simulink model "P1_Sim_2_1"  (R2021a)
settings: Solver=ode5  StartTime=0  StopTime=t  FixedStep=0.01  RelTol=1e-3  AbsTol=1e-6
model workspace (MAT data in the model file):
  socvcb = containers.Map
  socvcb.serialization.keys = {}
  socvcb.serialization.values = {}
  socvcb.serialization.uniformity = 0
  socvcb.serialization.keyType = 'double'
  socvcb.serialization.valueType = 'any'
values from neighbouring files (symbols this model uses):
  amplitude = 0.7    [control.m]
  g = 9.81    [control.m]
  gamma2 = 0.267534    [control.m]
  init_cond = [0 pi/30 0 0]    [control.m]
  K = lqr(A,B,Q,R)    [control.m]
  l = 0.512166    [control.m]
  M = 0.5723    [control.m]
  m = 0.12    [control.m]
  stab_point = [0 0 0 0]    [control.m]
libraries: simulink x12, pid_lib x3, simulink_extras x1
settings Model: ExtModeTrigDuration=18000  ExtModeTrigLevel=0.400000  Creator=jims  LastModifiedBy=Piotr
settings SolverCC: AutoScaleAbsTol=off  AlgebraicLoopSolver=TrustRegion
settings DataIOCC: ExternalInput=[]  InitialState=[]  MaxDataPoints=5000  SaveFormat=StructureWithTime  SignalLoggingSaveFormat=ModelDataLogs  SaveOutput=off  SaveTime=off  ReturnWorkspaceOutputs=off
settings OptimizationCC: BlockReduction=off  BooleanDataType=off  BufferReuse=off  ExpressionDepthLimit=2147483647
settings DebuggingCC: AlgebraicLoopMsg=none  SaveWithParameterizedLinksMsg=none  UnderspecifiedInitializationDetection=Classic  MergeDetectMultiDrivingBlocksExec=none  SignalResolutionControl=TryResolveAllWithWarning  MultiTaskDSMMsg=warning  MultiTaskCondExecSysMsg=none  IntegerOverflowMsg=none  FcnCallInpInsideContextMsg=warning  UnconnectedInputMsg=none  UnconnectedOutputMsg=none  UnconnectedLineMsg=none  StateNameClashWarn=warning  SFUnexpectedBacktrackingDiag=warning  SFNoUnconditionalDefaultTransitionDiag=warning  SFExecutionAtInitializationDiag=none  SFMachineParentedDataDiag=warning  IntegerSaturationMsg=none  ArithmeticOperatorsInVariantConditions=warning
settings HardwareCC: TargetBitPerLong=64  TargetBitPerPointer=64  TargetIntDivRoundTo=Zero  TargetEndianess=LittleEndian  TargetWordSize=64  TargetHWDeviceType=Intel->x86-64
settings ModelReferenceCC: PropagateSignalLabelsOutOfModel=off
settings SFSimCC: SimUseLocalCustomCode=off  CustomCodeUndefinedFunction=UseInterfaceOnly
settings RTWCC: Description=Generic Real-Time Target  RTWUseLocalCustomCode=off  RTWCompilerOptimization=on
settings CodeAppCC: MaxIdLength=95  StateflowObjectComments=on
settings GRTTargetCC: TargetLangStandard=C89/C90 (ANSI)
settings ConfigComp: CovMetricSettings=dw  CovSaveCumulativeToWorkspaceVar=on  CovSaveSingleToWorkspaceVar=on  CovExternalEMLEnable=off  CovSFcnEnable=off

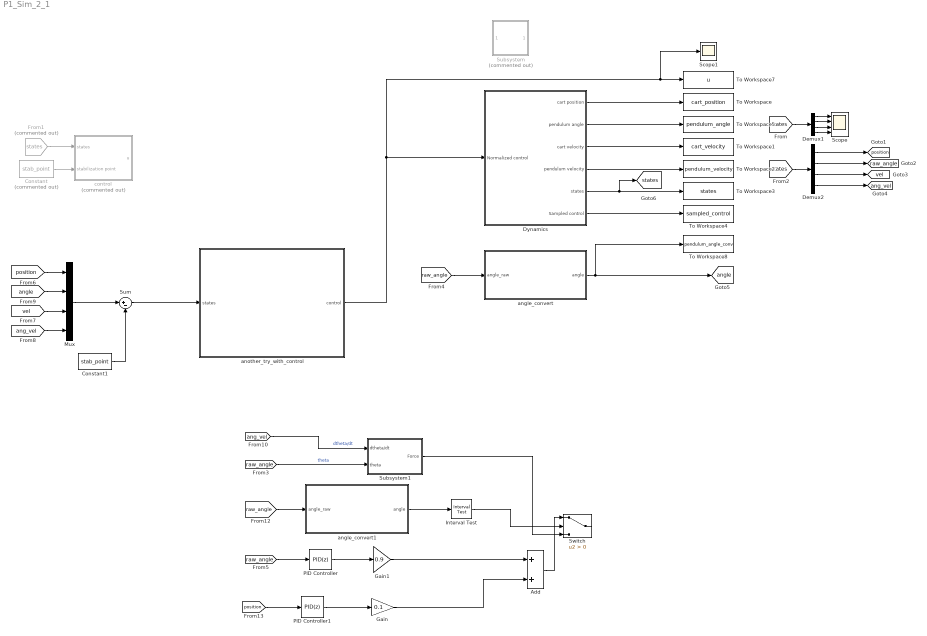
== system P1_Sim_2_1 ==
  Add : Sum
  Constant : Constant  Commented=on  Value=stab_point  OutDataTypeStr=Inherit: Inherit via back propagation
  Constant1 : Constant  Value=stab_point  OutDataTypeStr=Inherit: Inherit via back propagation
  Demux1 : Demux
  Demux2 : Demux
  Dynamics : Subsystem  mask(Dynamics){x_ini=init_cond, m=[0.5723, 0.12], fr=[0.00027344,  1.1975875,  0.5], P4=[0.01955717, 0.0038583, 9.81], Up=[ 12.86, 0.093125], DZ=[0.1, 1.5]}
      mask prompts: x_ini "Initial state vector [x1(0)  x2(0)  x3(0)  x4(0)]"; m "mass of cart (mc)  mass of pendulum (mp)"; fr "friction :  fp  FS  FC"; P4 "Distance (l), Total Inertia moment (J), gravity (g)"; Up "control : magnitude (M)    DZu"; DZ "minimal velocities : cart (DZcv)  pendulum (DZcp)"
      mask help:
      | Pendulum-Cart Dynamics
      |
      | Copyright INTECO 1997
      mask init:
      | DZcv=DZ(1);DZcp=DZ(2);DZu=Up(2);l=P4(1);J=P4(2);g=P4(3);M=Up(1);mc=m(1);mp=m(2);fp=fr(1);FS=fr(2);FC=fr(3);mi=l*(mc+mp);a=l*l+J/(mc+mp);
      mask Display: plot(0,0,100,100,[40,48,48,40,40],[60,60,49,49,60],[37,44],[9,54],[100,8,4,1,0,100,100,0,40,100,100,0,0,40],[44,44,44,44,45,46,45,44,45,45,43,43,46,46],[100,48],[55,55],[0,40],[55,55])
  From1 : From  Commented=on  GotoTag=states  TagVisibility=global
  Gain : Gain  Gain=0.1
  Gain1 : Gain  Gain=0.9
  Interval Test : simulink/Logic and Bit Operations/Interval Test  IntervalClosedRight=on  uplimit=0.5  IntervalClosedLeft=on  lowlimit=-0.5  OutDataTypeStr=boolean
  Mux : Mux
  PID Controller : pid_lib/PID Controller  Controller=PID  Form=Parallel  TimeDomain=Discrete-time  UseExternalTs=off  SampleTime=-1  IntegratorMethod=Forward Euler  FilterMethod=Forward Euler  ControllerParametersSource=internal  P=100  I=1  D=20  UseFilter=on  N=100  TunerSelectOption=Transfer Function Based (PID Tuner App)  InitialConditionSource=internal  InitialConditionForIntegrator=0  InitialConditionForFilter=0  DifferentiatorICPrevScaledInput=0  ExternalReset=none  TrackingMode=off  Kt=1  LimitOutput=off  SatLimitsSource=internal  UpperSaturationLimit=inf  LowerSaturationLimit=-inf  LinearizeAsGain=on  AntiWindupMode=none  Kb=1  POutMin=[]  POutMax=[]  IOutMin=[]  IOutMax=[]  DOutMin=[]  DOutMax=[]  NOutMin=[]  NOutMax=[]  SumOutMin=[]  SumOutMax=[]  SaturationOutMin=[]  SaturationOutMax=[]  PParamMin=[]  PParamMax=[]  IParamMin=[]  IParamMax=[]  DParamMin=[]  DParamMax=[]  NParamMin=[]  NParamMax=[]  KbParamMin=[]  KbParamMax=[]  KtParamMin=[]  KtParamMax=[]  KbOutMin=[]  KbOutMax=[]  KtOutMin=[]  KtOutMax=[]  IntegratorOutMin=[]  IntegratorOutMax=[]  FilterOutMin=[]  FilterOutMax=[]  SumI1OutMin=[]  SumI1OutMax=[]  SumI2OutMin=[]  SumI2OutMax=[]  SumI3OutMin=[]  SumI3OutMax=[]  SumI4OutMin=[]  SumI4OutMax=[]  SumDOutMin=[]  SumDOutMax=[]  DifferentiatorOutMin=[]  DifferentiatorOutMax=[]  FilterDiffOutCoefMin=[]  FilterDiffOutCoefMax=[]  ReciprocalOutMin=[]  ReciprocalOutMax=[]  SumDenOutMin=[]  SumDenOutMax=[]  SumNumOutMin=[]  SumNumOutMax=[]  DivideOutMin=[]  DivideOutMax=[]  UdiffTsProdOutMin=[]  UdiffTsProdOutMax=[]  NTsProdOutMin=[]  NTsProdOutMax=[]  UintegralTsProdOutMin=[]  UintegralTsProdOutMax=[]  UngainTsProdOutMin=[]  UngainTsProdOutMax=[]  IntegratorContinuousStateAttributes=''  IntegratorStateMustResolveToSignalObject=off  IntegratorRTWStateStorageClass=Auto  FilterContinuousStateAttributes=''  FilterStateMustResolveToSignalObject=off  FilterRTWStateStorageClass=Auto  ParallelPVariant=InternalParameters  IdealPVariant=Disabled  IVariant=InternalParameters  DVariant=InternalParameters  IntegratorVariant=Discrete  SatVariant=Disabled  AWVariant=Passthrough  PCopyVariant=Disabled  TRVariant=Disabled  FdbkBlocksVariant=Forward  IdealPFdbkVariant=Disabled  SatFdbkVariant=Disabled  DerivativeFilterVariant=ForwardEulerFilter  NVariant=InternalParameters  NCopyVariant=Disabled  FilterICVariant=InternalICsFilter  IntegratorICVariant=InternalICs  ExternalResetVariant=Disabled  TRSumVariant=Passthrough  SumFdbkVariant=Disabled  SumVariant=Sum_PID  TsampFilterVariant=InternalTs  TsampNgainVariant=Passthrough  TsampIntegralVariant=Passthrough  ExternalSaturationOutDataTypeStr=Inherit: Same as second input
  PID Controller1 : pid_lib/PID Controller  Controller=PID  Form=Parallel  TimeDomain=Discrete-time  UseExternalTs=off  SampleTime=-1  IntegratorMethod=Forward Euler  FilterMethod=Forward Euler  ControllerParametersSource=internal  P=100  I=1  D=20  UseFilter=on  N=100  TunerSelectOption=Transfer Function Based (PID Tuner App)  InitialConditionSource=internal  InitialConditionForIntegrator=0  InitialConditionForFilter=0  DifferentiatorICPrevScaledInput=0  ExternalReset=none  TrackingMode=off  Kt=1  LimitOutput=off  SatLimitsSource=internal  UpperSaturationLimit=inf  LowerSaturationLimit=-inf  LinearizeAsGain=on  AntiWindupMode=none  Kb=1  POutMin=[]  POutMax=[]  IOutMin=[]  IOutMax=[]  DOutMin=[]  DOutMax=[]  NOutMin=[]  NOutMax=[]  SumOutMin=[]  SumOutMax=[]  SaturationOutMin=[]  SaturationOutMax=[]  PParamMin=[]  PParamMax=[]  IParamMin=[]  IParamMax=[]  DParamMin=[]  DParamMax=[]  NParamMin=[]  NParamMax=[]  KbParamMin=[]  KbParamMax=[]  KtParamMin=[]  KtParamMax=[]  KbOutMin=[]  KbOutMax=[]  KtOutMin=[]  KtOutMax=[]  IntegratorOutMin=[]  IntegratorOutMax=[]  FilterOutMin=[]  FilterOutMax=[]  SumI1OutMin=[]  SumI1OutMax=[]  SumI2OutMin=[]  SumI2OutMax=[]  SumI3OutMin=[]  SumI3OutMax=[]  SumI4OutMin=[]  SumI4OutMax=[]  SumDOutMin=[]  SumDOutMax=[]  DifferentiatorOutMin=[]  DifferentiatorOutMax=[]  FilterDiffOutCoefMin=[]  FilterDiffOutCoefMax=[]  ReciprocalOutMin=[]  ReciprocalOutMax=[]  SumDenOutMin=[]  SumDenOutMax=[]  SumNumOutMin=[]  SumNumOutMax=[]  DivideOutMin=[]  DivideOutMax=[]  UdiffTsProdOutMin=[]  UdiffTsProdOutMax=[]  NTsProdOutMin=[]  NTsProdOutMax=[]  UintegralTsProdOutMin=[]  UintegralTsProdOutMax=[]  UngainTsProdOutMin=[]  UngainTsProdOutMax=[]  IntegratorContinuousStateAttributes=''  IntegratorStateMustResolveToSignalObject=off  IntegratorRTWStateStorageClass=Auto  FilterContinuousStateAttributes=''  FilterStateMustResolveToSignalObject=off  FilterRTWStateStorageClass=Auto  ParallelPVariant=InternalParameters  IdealPVariant=Disabled  IVariant=InternalParameters  DVariant=InternalParameters  IntegratorVariant=Discrete  SatVariant=Disabled  AWVariant=Passthrough  PCopyVariant=Disabled  TRVariant=Disabled  FdbkBlocksVariant=Forward  IdealPFdbkVariant=Disabled  SatFdbkVariant=Disabled  DerivativeFilterVariant=ForwardEulerFilter  NVariant=InternalParameters  NCopyVariant=Disabled  FilterICVariant=InternalICsFilter  IntegratorICVariant=InternalICs  ExternalResetVariant=Disabled  TRSumVariant=Passthrough  SumFdbkVariant=Disabled  SumVariant=Sum_PID  TsampFilterVariant=InternalTs  TsampNgainVariant=Passthrough  TsampIntegralVariant=Passthrough  ExternalSaturationOutDataTypeStr=Inherit: Same as second input
  Scope : Scope  NumInputPorts=4
  Scope1 : Scope
  Subsystem : Subsystem  Commented=on
  Subsystem1 : Subsystem
  Sum : Sum  Inputs=|+-
  Switch : Switch  Criteria=u2 > Threshold
  To Workspace : ToWorkspace  VariableName=cart_position  SampleTime=-1
  To Workspace1 : ToWorkspace  VariableName=cart_velocity  SampleTime=-1
  To Workspace2 : ToWorkspace  VariableName=pendulum_velocity  SampleTime=-1
  To Workspace3 : ToWorkspace  VariableName=states  SampleTime=-1
  To Workspace4 : ToWorkspace  VariableName=sampled_control  SampleTime=-1
  To Workspace5 : ToWorkspace  VariableName=pendulum_angle  SampleTime=-1
  To Workspace7 : ToWorkspace  VariableName=u  SampleTime=-1
  To Workspace8 : ToWorkspace  VariableName=pendulum_angle_conv  SampleTime=-1
  angle_convert : MATLAB Function  TreatAsAtomicUnit=on
  angle_convert1 : MATLAB Function  TreatAsAtomicUnit=on
  another_try_with_control : Subsystem
  control : Subsystem  Commented=on
  tag scope: ang_vel=global, angle=global, position=global, raw_angle=global, states=global, vel=global
  wires:
  Dynamics/1(cart position) -> To Workspace/1
  Dynamics/6(Sampled control) -> To Workspace4/1
  Dynamics/4(pendulum velocity) -> To Workspace2/1
  Dynamics/3(cart velocity) -> To Workspace1/1
  Demux1/1 -> Scope/1
  Demux1/2 -> Scope/2
  Demux1/3 -> Scope/3
  Demux1/4 -> Scope/4
  [states] -> Demux1/1
  [states] -> Demux2/1
  Demux2/1 -> [position]
  Demux2/2 -> [raw_angle]
  Demux2/3 -> [vel]
  Demux2/4 -> [ang_vel]
  Constant/1 -> control/2(stabilization point)
  [raw_angle] -> angle_convert/1(angle_raw)
  angle_convert/1(angle) -> [angle], To Workspace8/1
  Dynamics/2(pendulum angle) -> To Workspace5/1
  Dynamics/5(states) -> [states], To Workspace3/1
  From1/1 -> control/1(states)
  Mux/1 -> Sum/1
  Constant1/1 -> Sum/2
  [position] -> Mux/1
  [vel] -> Mux/3
  [angle] -> Mux/2
  [ang_vel] -> Mux/4
  Sum/1 -> another_try_with_control/1(states)
  another_try_with_control/1(control) -> Dynamics/1(Normalized control), Scope1/1, To Workspace7/1
  Subsystem1/1(Force) -> Switch/3
  Gain/1 -> Add/2
  Add/1 -> Switch/1
  Interval Test/1 -> Switch/2
  [position] -> PID Controller1/1
  PID Controller/1 -> Gain1/1
  Gain1/1 -> Add/1
  angle_convert1/1(angle) -> Interval Test/1
  PID Controller1/1 -> Gain/1
  [raw_angle] -> Subsystem1/2(theta)  "theta"
  [ang_vel] -> Subsystem1/1(dtheta/dt)  "dtheta/dt"
  [raw_angle] -> angle_convert1/1(angle_raw)
  [raw_angle] -> PID Controller/1

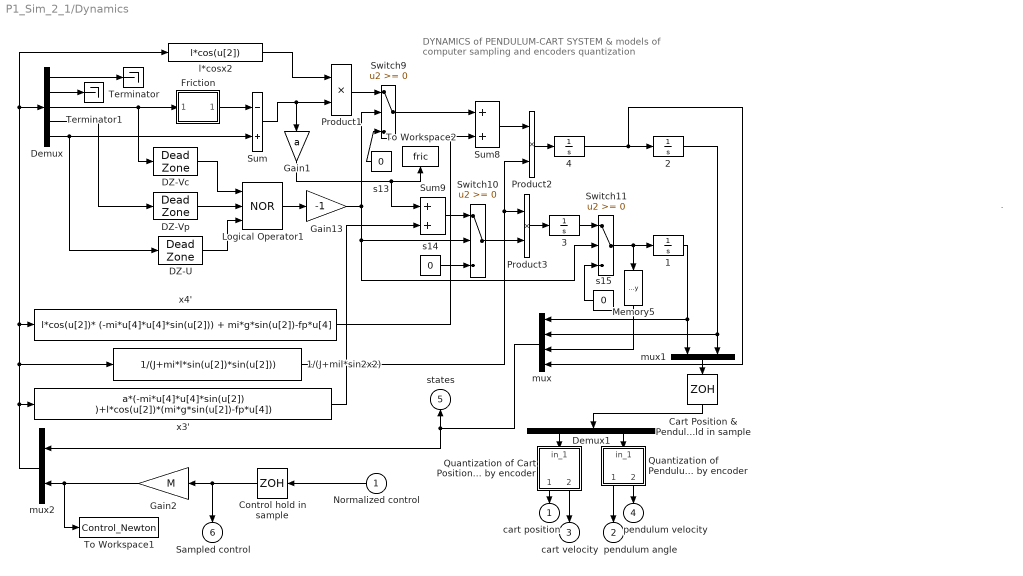
== system P1_Sim_2_1/Dynamics ==
  note: DYNAMICS of
      | PENDULUM-CART SYSTEM
      | & models of
      | computer sampling and encoders quantization
  note: .
  Normalized control : Inport
  " Quantization of Pendulum Angle introduced by encoder" : Subsystem
  1 : Integrator  InitialCondition=x_ini(1)
  1/(J+mil*sin2x2) : Fcn  Expr=1/(J+mi*l*sin(u[2])*sin(u[2]))
  2 : Integrator  InitialCondition=x_ini(2)
  3 : Integrator  InitialCondition=x_ini(3)
  4 : Integrator  InitialCondition=x_ini(4)
  Cart Position & Pendulum Angle hold in sample : ZeroOrderHold  SampleTime=0.01
  Control hold in sample : ZeroOrderHold  SampleTime=0.01
  DZ-U : DeadZone  LowerValue=-DZu  UpperValue=DZu  SaturateOnIntegerOverflow=on
  DZ-Vc : DeadZone  LowerValue=-DZcv  UpperValue=DZcv  SaturateOnIntegerOverflow=on
  DZ-Vp : DeadZone  LowerValue=-DZcp  UpperValue=DZcp  SaturateOnIntegerOverflow=on
  Demux : Demux  Outputs=5
      settings: DisplayOption=none
  Demux1 : Demux  Outputs=2
      settings: DisplayOption=none
  Friction : Subsystem  mask(Coulombic and Viscous Friction){FS=FS, FC=FC}
      mask prompts: FS "Static friction"; FC "Coulomb friction"
      mask help:
      | A discontinuity offset at zero models coulomb friction.  Linear gain models viscous friction.
      | y = sign(x) * (Umax * abs(x) + friction)
      mask Help:
      | This block has a discontinuity
      | at zero and a linear gain afterward.
      | y= sign(x)*(Umax*abs(x)+friction)
  Gain1 : Gain  Gain=a  SaturateOnIntegerOverflow=on  OutDataTypeStr=Inherit: Same as input  ParamDataTypeStr=Inherit: Same as input
  Gain13 : Gain  Gain=-1  SaturateOnIntegerOverflow=on  OutDataTypeStr=Inherit: Same as input  ParamDataTypeStr=Inherit: Same as input
  Gain2 : Gain  Gain=M  SaturateOnIntegerOverflow=on  OutDataTypeStr=Inherit: Same as input  ParamDataTypeStr=Inherit: Same as input
  Logical Operator1 : Logic  Operator=NOR  Inputs=3
  Memory5 : Memory
  Product1 : Product  InputSameDT=on  RndMeth=Zero  SaturateOnIntegerOverflow=on  OutDataTypeStr=Inherit: Same as first input
  Product2 : Product  InputSameDT=on  RndMeth=Zero  SaturateOnIntegerOverflow=on  OutDataTypeStr=Inherit: Same as first input
  Product3 : Product  InputSameDT=on  RndMeth=Zero  SaturateOnIntegerOverflow=on  OutDataTypeStr=Inherit: Same as first input
  "Quantization of Cart Position introduced by encoder " : Subsystem
  Sum : Sum  Inputs=-+  InputSameDT=on  SaturateOnIntegerOverflow=on  OutDataTypeStr=Inherit: Same as first input
  Sum8 : Sum  InputSameDT=on  SaturateOnIntegerOverflow=on  OutDataTypeStr=Inherit: Same as first input
  Sum9 : Sum  InputSameDT=on  SaturateOnIntegerOverflow=on  OutDataTypeStr=Inherit: Same as first input
  Switch10 : Switch  SaturateOnIntegerOverflow=on  InputSameDT=on
  Switch11 : Switch  SaturateOnIntegerOverflow=on  InputSameDT=on
  Switch9 : Switch  SaturateOnIntegerOverflow=on  InputSameDT=on
  Terminator : Terminator
  Terminator1 : Terminator
  To Workspace1 : ToWorkspace  VariableName=Control_Newton
      settings: MaxDataPoints=100000
  To Workspace2 : ToWorkspace  VariableName=fric
      settings: MaxDataPoints=100000
  l*cosx2 : Fcn  Expr=l*cos(u[2])
  mux : Mux
  mux1 : Mux  Inputs=2
  mux2 : Mux  Inputs=[4 1]
  s13 : Constant  Value=0
  s14 : Constant  Value=0
  s15 : Constant  Value=0
  x3' : Fcn  Expr=a*(-mi*u[4]*u[4]*sin(u[2]) )+l*cos(u[2])*(mi*g*sin(u[2])-fp*u[4])
  x4' : Fcn  Expr=l*cos(u[2])* (-mi*u[4]*u[4]*sin(u[2])) + mi*g*sin(u[2])-fp*u[4]
  cart position : Outport  InitialOutput=0
  pendulum angle : Outport  Port=2  InitialOutput=0
  cart velocity : Outport  Port=3  InitialOutput=0
  pendulum velocity : Outport  Port=4  InitialOutput=0
  states : Outport  Port=5  InitialOutput=0
  Sampled control : Outport  Port=6  InitialOutput=0
  wires:
  Demux1/1 -> "Quantization of Cart Position introduced by encoder "/1(in_1)
  mux/1 -> mux2/1, states/1
  "Quantization of Cart Position introduced by encoder "/1(out_1) -> cart position/1
  "Quantization of Cart Position introduced by encoder "/2(out_2) -> cart velocity/1
  " Quantization of Pendulum Angle introduced by encoder"/2(out_2) -> pendulum velocity/1
  Demux1/2 -> " Quantization of Pendulum Angle introduced by encoder"/1(in_1)
  Control hold in sample/1 -> Sampled control/1, Gain2/1
  Normalized control/1 -> Control hold in sample/1
  Cart Position & Pendulum Angle hold in sample/1 -> Demux1/1
  mux1/1 -> Cart Position & Pendulum Angle hold in sample/1
  4/1 -> mux/4, 2/1
  Switch11/1 -> Memory5/1, 1/1
  Memory5/1 -> mux/3
  Demux/2 -> Terminator1/1
  Demux/5 -> DZ-U/1, Sum/2
  Demux/1 -> Terminator/1
  Demux/4 -> DZ-Vp/1
  Demux/3 -> DZ-Vc/1, Friction/1(In1)
  DZ-U/1 -> Logical Operator1/3
  Logical Operator1/1 -> Gain13/1
  DZ-Vp/1 -> Logical Operator1/2
  DZ-Vc/1 -> Logical Operator1/1
  l*cosx2/1 -> Product1/1
  s13/1 -> Switch9/3
  Switch9/1 -> Sum8/1
  s14/1 -> Switch10/3
  Product1/1 -> Switch9/1
  x4'/1 -> Sum8/2
  Sum8/1 -> Product2/1
  Product2/1 -> 4/1
  Product3/1 -> 3/1
  Sum9/1 -> Switch10/1
  3/1 -> Switch11/1
  s15/1 -> Switch11/3
  Gain13/1 -> Switch9/2, Switch11/2, Switch10/2
  Switch10/1 -> Product3/2
  Sum/1 -> Product1/2, Gain1/1
  mux2/1 -> x3'/1, Demux/1, l*cosx2/1, x4'/1, 1/(J+mil*sin2x2)/1
  1/(J+mil*sin2x2)/1 -> Product2/2, Product3/1
  Gain1/1 -> Sum9/1, To Workspace2/1
  Gain2/1 -> To Workspace1/1, mux2/2
  Friction/1(Out1) -> Sum/1
  " Quantization of Pendulum Angle introduced by encoder"/1(out_1) -> pendulum angle/1
  2/1 -> mux/2, mux1/2
  x3'/1 -> Sum9/2
  1/1 -> mux/1, mux1/1

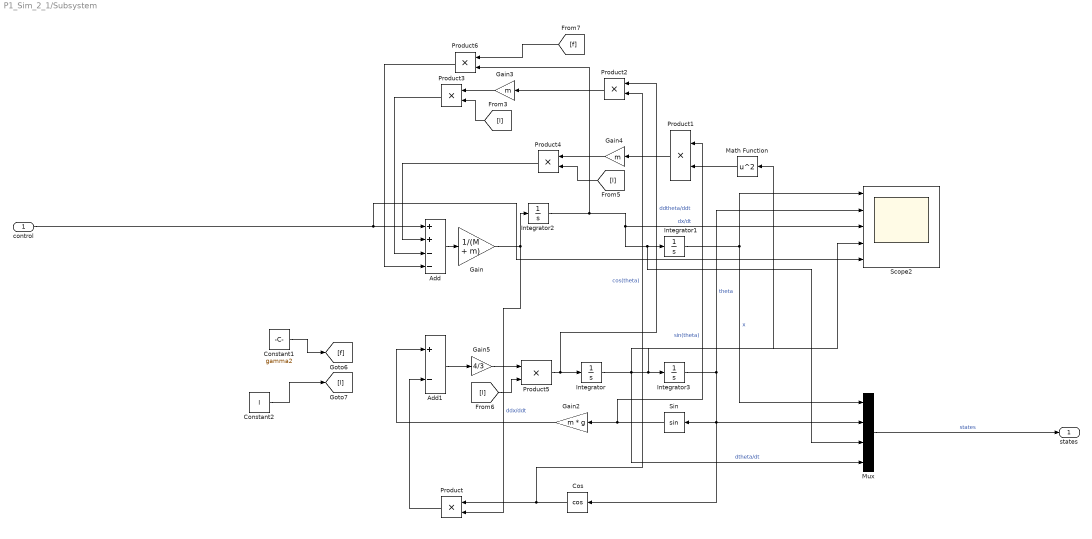
== system P1_Sim_2_1/Subsystem ==
  control : Inport
  Add : Sum  Inputs=++--
  Add1 : Sum  Inputs=+-
  Constant1 : Constant  Value=gamma2
  Constant2 : Constant  Value=l
  Cos : Trigonometry  Operator=cos
  Gain : Gain  Gain=1/(M + m)
  Gain2 : Gain  Gain=m * g
  Gain3 : Gain  Gain=m
  Gain4 : Gain  Gain=m
  Gain5 : Gain  Gain=4/3
  Integrator : Integrator  InitialCondition=init_cond(4)
  Integrator1 : Integrator  InitialCondition=init_cond(1)
  Integrator2 : Integrator  InitialCondition=init_cond(3)
  Integrator3 : Integrator  InitialCondition=init_cond(2)
  Math Function : Math  Operator=square  SaturateOnIntegerOverflow=on
  Mux : Mux
  Product{,1..6} (7 alike) : Product
  Scope2 : Scope  NumInputPorts=5
  Sin : Trigonometry
  states : Outport
  wires:
  Integrator3/1 -> Scope2/2, Cos/1, Sin/1, Mux/2  "theta"
  Gain2/1 -> Add1/1
  Constant2/1 -> [l]
  control/1 -> Scope2/5, Add/1
  Product5/1 -> Product2/1, Integrator/1  "ddtheta/ddt"
  Math Function/1 -> Product1/2
  Integrator2/1 -> Mux/3, Integrator1/1, Scope2/3, Product6/2  "dx/dt"
  Product4/1 -> Add/2
  Integrator1/1 -> Mux/1, Scope2/1  "x"
  Add/1 -> Gain/1
  Constant1/1 -> [f]
  [l] -> Product4/2
  Product6/1 -> Add/4
  [f] -> Product6/1
  Gain5/1 -> Product5/1
  [l] -> Product5/2
  Product2/1 -> Gain3/1
  Product1/1 -> Gain4/1
  Gain/1 -> Product/2, Integrator2/1  "ddx/ddt"
  Cos/1 -> Product2/2, Product/1  "cos(theta)"
  Gain3/1 -> Product3/1
  Integrator/1 -> Scope2/4, Math Function/1, Integrator3/1, Mux/4  "dtheta/dt"
  Product3/1 -> Add/3
  Add1/1 -> Gain5/1
  [l] -> Product3/2
  Gain4/1 -> Product4/1
  Product/1 -> Add1/2
  Sin/1 -> Gain2/1, Product1/1  "sin(theta)"
  Mux/1 -> states/1  "states"

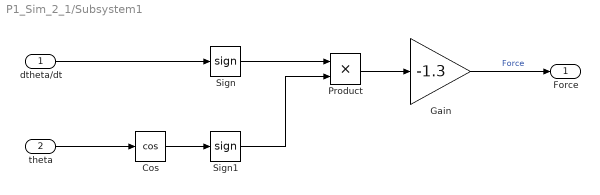
== system P1_Sim_2_1/Subsystem1 ==
  dtheta/dt : Inport
  theta : Inport  Port=2
  Cos : Trigonometry  Operator=cos
  Gain : Gain  Gain=-1.3
  Product : Product
  Sign : Signum
  Sign1 : Signum
  Force : Outport
  wires:
  Cos/1 -> Sign1/1
  Product/1 -> Gain/1
  Sign1/1 -> Product/2
  Gain/1 -> Force/1  "Force"
  Sign/1 -> Product/1
  theta/1 -> Cos/1
  dtheta/dt/1 -> Sign/1

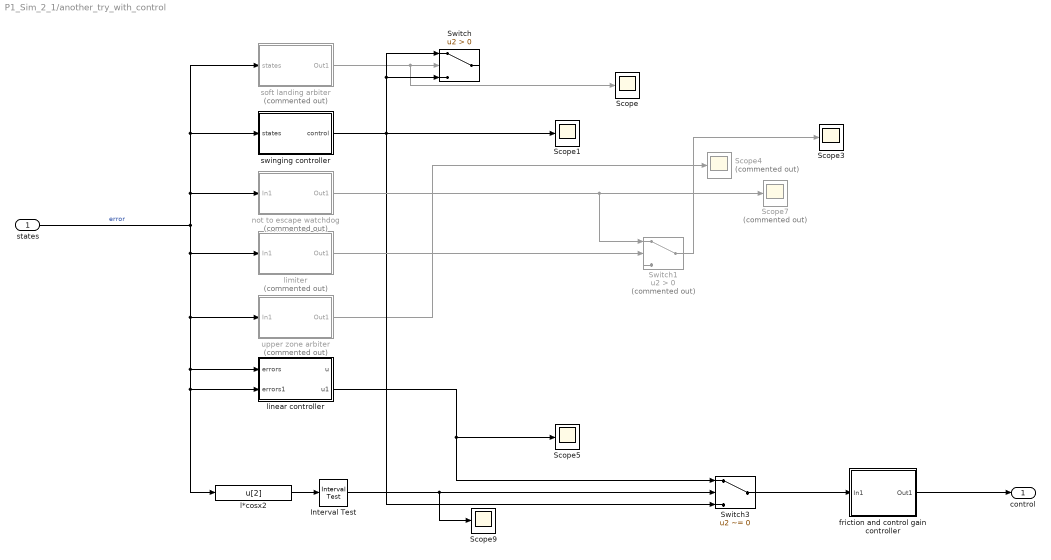
== system P1_Sim_2_1/another_try_with_control ==
  states : Inport
  Interval Test : simulink/Logic and Bit Operations/Interval Test  IntervalClosedRight=on  uplimit=pi/20  IntervalClosedLeft=on  lowlimit=-pi/20  OutDataTypeStr=boolean
  Scope{,1,3,5,9} (5 alike) : Scope
  Scope4 : Scope  Commented=on
  Scope7 : Scope  Commented=on
  Switch : Switch  Criteria=u2 > Threshold
  Switch1 : Switch  Commented=on  Criteria=u2 > Threshold
  Switch3 : Switch  Criteria=u2 ~= 0
  friction and control gain controller : Subsystem
  l*cosx2 : Fcn  Expr=u[2]
  limiter : Subsystem  Commented=on
  linear controller : Subsystem
  not to escape watchdog : Subsystem  Commented=on
  soft landing arbiter : Subsystem  Commented=on
  swinging controller : Subsystem
  upper zone arbiter : Subsystem  Commented=on
  control : Outport
  wires:
  states/1 -> l*cosx2/1, linear controller/2(errors1), linear controller/1(errors), upper zone arbiter/1(In1), limiter/1(In1), soft landing arbiter/1(states), swinging controller/1(states), not to escape watchdog/1(In1)  "error"
  soft landing arbiter/1(Out1) -> Scope/1, Switch/2
  upper zone arbiter/1(Out1) -> Scope4/1
  linear controller/2(u1) -> Switch3/1, Scope5/1
  swinging controller/1(control) -> Switch/1, Switch/3, Scope1/1, Switch3/3
  limiter/1(Out1) -> Switch1/2
  not to escape watchdog/1(Out1) -> Switch1/1, Scope7/1
  Switch1/1 -> Scope3/1
  Interval Test/1 -> Scope9/1, Switch3/2
  Switch3/1 -> friction and control gain controller/1(In1)
  l*cosx2/1 -> Interval Test/1
  friction and control gain controller/1(Out1) -> control/1

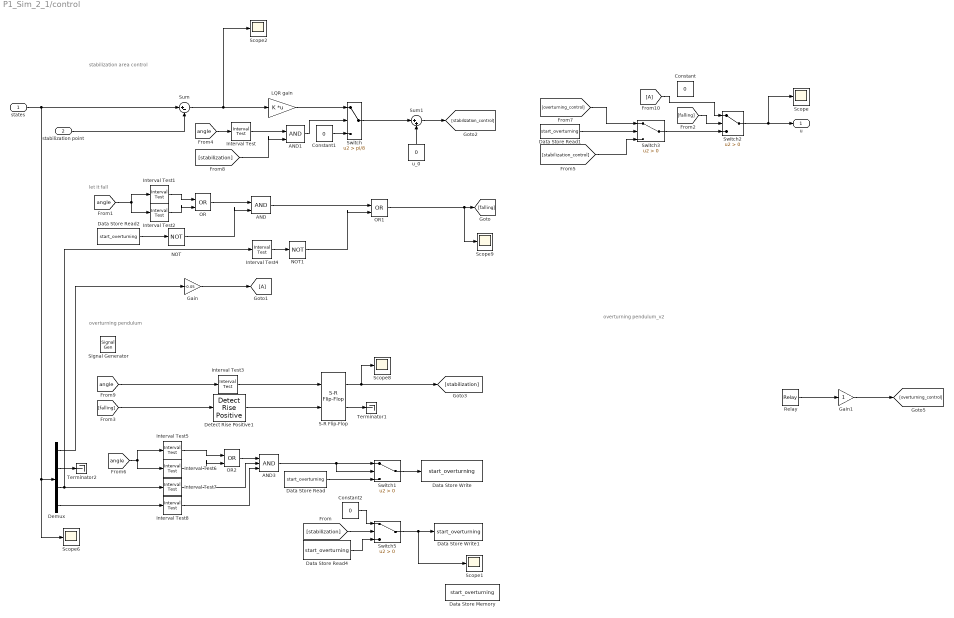
== system P1_Sim_2_1/control ==
  note: overturning pendulum
  note: stabilization area control
  note: let it fall
  note: overturning pendulum_v2
  states : Inport
  stabilization point : Inport  Port=2
  AND : Logic  IconShape=distinctive  AllPortsSameDT=off  OutDataTypeStr=boolean
  AND1 : Logic  IconShape=distinctive  AllPortsSameDT=off  OutDataTypeStr=boolean
  AND3 : Logic  Inputs=3  IconShape=distinctive  AllPortsSameDT=off  OutDataTypeStr=boolean
  Constant : Constant  Value=0
  Constant1 : Constant  Value=0
  Constant2 : Constant  Value=0
  Data Store Memory : DataStoreMemory  DataStoreName=start_overturning  ShowAdditionalParam=off
  Data Store Read{,1..2,4} (4 alike) : DataStoreRead  DataStoreName=start_overturning  IndexOptions=Index vector (dialog)  Indices=1  OutputSizes=1
  Data Store Write : DataStoreWrite  DataStoreName=start_overturning  IndexOptions=Index vector (dialog)  Indices=1  OutputSizes=1
  Data Store Write1 : DataStoreWrite  DataStoreName=start_overturning  IndexOptions=Index vector (dialog)  Indices=1  OutputSizes=1
  Demux : Demux
  Detect Rise Positive1 : simulink/Logic and Bit Operations/Detect Rise Positive  vinit=0  OutDataTypeStr=boolean
  Gain : Gain  Gain=-0.05
  Gain1 : Gain
  Interval Test : simulink/Logic and Bit Operations/Interval Test  IntervalClosedRight=off  uplimit=pi/90  IntervalClosedLeft=off  lowlimit=-pi/90  OutDataTypeStr=boolean
  Interval Test1 : simulink/Logic and Bit Operations/Interval Test  IntervalClosedRight=on  uplimit=pi  IntervalClosedLeft=on  lowlimit=pi/8  OutDataTypeStr=boolean
  Interval Test2 : simulink/Logic and Bit Operations/Interval Test  IntervalClosedRight=on  uplimit=-pi/8  IntervalClosedLeft=on  lowlimit=-pi  OutDataTypeStr=boolean
  Interval Test3 : simulink/Logic and Bit Operations/Interval Test  IntervalClosedRight=on  uplimit=pi/90  IntervalClosedLeft=on  lowlimit=-pi/90  OutDataTypeStr=boolean
  Interval Test4 : simulink/Logic and Bit Operations/Interval Test  IntervalClosedRight=on  uplimit=20  IntervalClosedLeft=on  lowlimit=-20  OutDataTypeStr=boolean
  Interval Test5 : simulink/Logic and Bit Operations/Interval Test  IntervalClosedRight=on  uplimit=pi  IntervalClosedLeft=on  lowlimit=14*pi/15  OutDataTypeStr=boolean
  Interval Test6 : simulink/Logic and Bit Operations/Interval Test  IntervalClosedRight=on  uplimit=-14*pi/15  IntervalClosedLeft=on  lowlimit=-pi  OutDataTypeStr=boolean
  Interval Test7 : simulink/Logic and Bit Operations/Interval Test  IntervalClosedRight=on  uplimit=0.1  IntervalClosedLeft=on  lowlimit=-0.1  OutDataTypeStr=boolean
  Interval Test8 : simulink/Logic and Bit Operations/Interval Test  IntervalClosedRight=on  uplimit=0.1  IntervalClosedLeft=on  lowlimit=-0.1  OutDataTypeStr=boolean
  LQR gain : Gain  Gain=K  Multiplication=Matrix(K*u)
  NOT : Logic  Operator=NOT  IconShape=distinctive  AllPortsSameDT=off  OutDataTypeStr=boolean
  NOT1 : Logic  Operator=NOT  IconShape=distinctive  AllPortsSameDT=off  OutDataTypeStr=boolean
  OR : Logic  Operator=OR  IconShape=distinctive  AllPortsSameDT=off  OutDataTypeStr=boolean
  OR1 : Logic  Operator=OR  IconShape=distinctive  AllPortsSameDT=off  OutDataTypeStr=boolean
  OR2 : Logic  Operator=OR  IconShape=distinctive  AllPortsSameDT=off  OutDataTypeStr=boolean
  Relay : Relay
  S-R Flip-Flop : simulink_extras/Flip Flops/S-R Flip-Flop  initial_condition=0
  Scope{,1..2,6,8..9} (6 alike) : Scope
  Signal Generator : SignalGenerator  WaveForm=square  Amplitude=amplitude  Frequency=10  Units=rad/sec
  Sum : Sum  Inputs=|+-
  Sum1 : Sum  Inputs=|++
  Switch : Switch  Criteria=u2 > Threshold  Threshold=pi/8
  Switch{1..3,5} (4 alike) : Switch  Criteria=u2 > Threshold
  Terminator1 : Terminator
  Terminator2 : Terminator
  u_0 : Constant  Value=0
  u : Outport
  wires:
  LQR gain/1 -> Switch/1
  Interval Test/1 -> AND1/1
  Sum/1 -> Scope2/1, LQR gain/1
  [angle] -> Interval Test/1
  Constant1/1 -> Switch/3
  u_0/1 -> Sum1/2
  Switch/1 -> Sum1/1
  stabilization point/1 -> Sum/2
  [angle] -> Interval Test2/1, Interval Test1/1
  Interval Test1/1 -> OR/1
  Interval Test2/1 -> OR/2
  [falling] -> Switch2/2
  Switch2/1 -> Scope/1, u/1
  Sum1/1 -> [stabilization_control]
  Switch3/1 -> Switch2/3
  OR/1 -> AND/1
  AND1/1 -> Switch/2
  [stabilization] -> AND1/2
  [angle] -> Interval Test3/1
  Interval Test3/1 -> S-R Flip-Flop/1
  S-R Flip-Flop/1 -> [stabilization], Scope8/1
  Demux/3 -> Interval Test4/1, Interval Test7/1
  Demux/4 -> Interval Test8/1
  Interval Test6/1 -> OR2/2
  Interval Test5/1 -> OR2/1
  OR2/1 -> AND3/1
  Interval Test7/1 -> AND3/2
  Interval Test8/1 -> AND3/3
  AND3/1 -> Switch1/1, Switch1/2
  [falling] -> Detect Rise Positive1/1
  Detect Rise Positive1/1 -> S-R Flip-Flop/2
  S-R Flip-Flop/2 -> Terminator1/1
  Data Store Read/1 -> Switch1/3
  Switch1/1 -> Data Store Write/1
  Data Store Read1/1 -> Switch3/2
  [stabilization_control] -> Switch3/3
  [overturning_control] -> Switch3/1
  [stabilization] -> Switch5/2
  Constant2/1 -> Switch5/1
  Data Store Read4/1 -> Switch5/3
  states/1 -> Scope6/1, Demux/1, Sum/1
  Data Store Read2/1 -> NOT/1
  NOT/1 -> AND/2
  Switch5/1 -> Scope1/1, Data Store Write1/1
  Demux/2 -> Terminator2/1
  [angle] -> Interval Test5/1, Interval Test6/1
  OR1/1 -> Scope9/1, [falling]
  AND/1 -> OR1/1
  NOT1/1 -> OR1/2
  Interval Test4/1 -> NOT1/1
  Demux/1 -> Gain/1
  Gain/1 -> [A]
  [A] -> Switch2/1
  Gain1/1 -> [overturning_control]
  Relay/1 -> Gain1/1

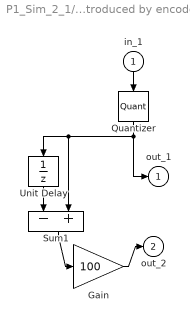
== system P1_Sim_2_1/Dynamics/ Quantization of Pendulum Angle introduced by encoder ==
  in_1 : Inport
  Gain : Gain  Gain=100  SaturateOnIntegerOverflow=on  OutDataTypeStr=Inherit: Same as input  ParamDataTypeStr=Inherit: Same as input
  Quantizer : Quantizer  QuantizationInterval=0.001534
  Sum1 : Sum  Inputs=-+  InputSameDT=on  SaturateOnIntegerOverflow=on  OutDataTypeStr=Inherit: Same as first input
  Unit Delay : UnitDelay  InitialCondition=x_ini(2)  SampleTime=0.01  HasFrameUpgradeWarning=on
  out_1 : Outport  InitialOutput=0
  out_2 : Outport  Port=2  InitialOutput=0
  wires:
  in_1/1 -> Quantizer/1
  Quantizer/1 -> Sum1/2, Unit Delay/1, out_1/1
  Sum1/1 -> Gain/1
  Gain/1 -> out_2/1
  Unit Delay/1 -> Sum1/1

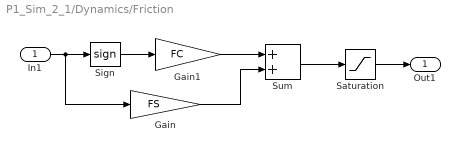
== system P1_Sim_2_1/Dynamics/Friction ==
  In1 : Inport
  Gain : Gain  Gain=FS  SaturateOnIntegerOverflow=on  OutDataTypeStr=Inherit: Same as input  ParamDataTypeStr=Inherit: Same as input
  Gain1 : Gain  Gain=FC  SaturateOnIntegerOverflow=on  OutDataTypeStr=Inherit: Same as input  ParamDataTypeStr=Inherit: Same as input
  Saturation : Saturate  UpperLimit=1  LowerLimit=-1
  Sign : Signum
  Sum : Sum  InputSameDT=on  SaturateOnIntegerOverflow=on  OutDataTypeStr=Inherit: Same as first input
  Out1 : Outport  InitialOutput=0
  wires:
  Saturation/1 -> Out1/1
  Sum/1 -> Saturation/1
  Sign/1 -> Gain1/1
  In1/1 -> Gain/1, Sign/1
  Gain1/1 -> Sum/1
  Gain/1 -> Sum/2

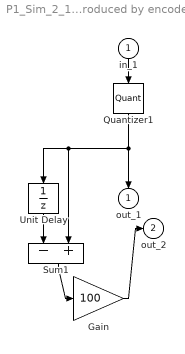
== system P1_Sim_2_1/Dynamics/Quantization of Cart Position introduced by encoder  ==
  in_1 : Inport
  Gain : Gain  Gain=100  SaturateOnIntegerOverflow=on  OutDataTypeStr=Inherit: Same as input  ParamDataTypeStr=Inherit: Same as input
  Quantizer1 : Quantizer  QuantizationInterval=5.7053e-005
  Sum1 : Sum  Inputs=-+  InputSameDT=on  SaturateOnIntegerOverflow=on  OutDataTypeStr=Inherit: Same as first input
  Unit Delay : UnitDelay  InitialCondition=x_ini(1)  SampleTime=0.01  HasFrameUpgradeWarning=on
  out_1 : Outport  InitialOutput=0
  out_2 : Outport  Port=2  InitialOutput=0
  wires:
  Quantizer1/1 -> Sum1/2, Unit Delay/1, out_1/1
  Unit Delay/1 -> Sum1/1
  Gain/1 -> out_2/1
  in_1/1 -> Quantizer1/1
  Sum1/1 -> Gain/1

== system P1_Sim_2_1/another_try_with_control/friction and control gain controller ==
  In1 : Inport
  Gain : Gain
  Saturation : Saturate  UpperLimit=1  LowerLimit=-1
  Sign : Signum
  Sum : Sum  Inputs=|++
  friction : Gain  Gain=0.05
  Out1 : Outport
  wires:
  In1/1 -> Gain/1, Sign/1
  Sign/1 -> friction/1
  friction/1 -> Sum/1
  Sum/1 -> Saturation/1
  Gain/1 -> Sum/2
  Saturation/1 -> Out1/1

== system P1_Sim_2_1/another_try_with_control/limiter ==
  In1 : Inport
  l*cosx2 : Fcn  Expr=abs(u[1]) - 1
  Out1 : Outport
  wires:
  In1/1 -> l*cosx2/1
  l*cosx2/1 -> Out1/1

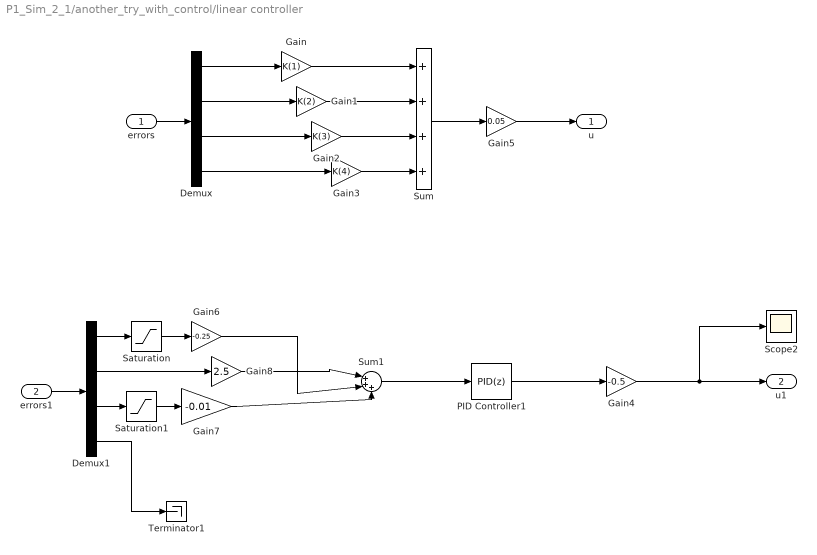
== system P1_Sim_2_1/another_try_with_control/linear controller ==
  errors : Inport
  errors1 : Inport  Port=2
  Demux : Demux
  Demux1 : Demux
  Gain : Gain  Gain=K(1)
  Gain1 : Gain  Gain=K(2)
  Gain2 : Gain  Gain=K(3)
  Gain3 : Gain  Gain=K(4)
  Gain4 : Gain  Gain=-0.5
  Gain5 : Gain  Gain=0.05
  Gain6 : Gain  Gain=-0.25
  Gain7 : Gain  Gain=-0.01
  Gain8 : Gain  Gain=2.5
  PID Controller1 : pid_lib/PID Controller  Controller=PID  Form=Parallel  TimeDomain=Discrete-time  UseExternalTs=off  SampleTime=0.01  IntegratorMethod=Forward Euler  FilterMethod=Forward Euler  ControllerParametersSource=internal  P=10  I=0.1  D=0.05  UseFilter=on  N=100  TunerSelectOption=Transfer Function Based (PID Tuner App)  InitialConditionSource=internal  InitialConditionForIntegrator=0  InitialConditionForFilter=0  DifferentiatorICPrevScaledInput=0  ExternalReset=none  TrackingMode=off  Kt=1  LimitOutput=off  SatLimitsSource=internal  UpperSaturationLimit=inf  LowerSaturationLimit=-inf  LinearizeAsGain=on  AntiWindupMode=none  Kb=1  POutMin=[]  POutMax=[]  IOutMin=[]  IOutMax=[]  DOutMin=[]  DOutMax=[]  NOutMin=[]  NOutMax=[]  SumOutMin=[]  SumOutMax=[]  SaturationOutMin=[]  SaturationOutMax=[]  PParamMin=[]  PParamMax=[]  IParamMin=[]  IParamMax=[]  DParamMin=[]  DParamMax=[]  NParamMin=[]  NParamMax=[]  KbParamMin=[]  KbParamMax=[]  KtParamMin=[]  KtParamMax=[]  KbOutMin=[]  KbOutMax=[]  KtOutMin=[]  KtOutMax=[]  IntegratorOutMin=[]  IntegratorOutMax=[]  FilterOutMin=[]  FilterOutMax=[]  SumI1OutMin=[]  SumI1OutMax=[]  SumI2OutMin=[]  SumI2OutMax=[]  SumI3OutMin=[]  SumI3OutMax=[]  SumI4OutMin=[]  SumI4OutMax=[]  SumDOutMin=[]  SumDOutMax=[]  DifferentiatorOutMin=[]  DifferentiatorOutMax=[]  FilterDiffOutCoefMin=[]  FilterDiffOutCoefMax=[]  ReciprocalOutMin=[]  ReciprocalOutMax=[]  SumDenOutMin=[]  SumDenOutMax=[]  SumNumOutMin=[]  SumNumOutMax=[]  DivideOutMin=[]  DivideOutMax=[]  UdiffTsProdOutMin=[]  UdiffTsProdOutMax=[]  NTsProdOutMin=[]  NTsProdOutMax=[]  UintegralTsProdOutMin=[]  UintegralTsProdOutMax=[]  UngainTsProdOutMin=[]  UngainTsProdOutMax=[]  IntegratorContinuousStateAttributes=''  IntegratorStateMustResolveToSignalObject=off  IntegratorRTWStateStorageClass=Auto  FilterContinuousStateAttributes=''  FilterStateMustResolveToSignalObject=off  FilterRTWStateStorageClass=Auto  ParallelPVariant=InternalParameters  IdealPVariant=Disabled  IVariant=InternalParameters  DVariant=InternalParameters  IntegratorVariant=Discrete  SatVariant=Disabled  AWVariant=Passthrough  PCopyVariant=Disabled  TRVariant=Disabled  FdbkBlocksVariant=Forward  IdealPFdbkVariant=Disabled  SatFdbkVariant=Disabled  DerivativeFilterVariant=ForwardEulerFilter  NVariant=InternalParameters  NCopyVariant=Disabled  FilterICVariant=InternalICsFilter  IntegratorICVariant=InternalICs  ExternalResetVariant=Disabled  TRSumVariant=Passthrough  SumFdbkVariant=Disabled  SumVariant=Sum_PID  TsampFilterVariant=InternalTs  TsampNgainVariant=Passthrough  TsampIntegralVariant=Passthrough  ExternalSaturationOutDataTypeStr=Inherit: Same as second input
  Saturation : Saturate  UpperLimit=0.4  LowerLimit=-0.4
  Saturation1 : Saturate  UpperLimit=2  LowerLimit=-2
  Scope2 : Scope
  Sum : Sum  Inputs=++++
  Sum1 : Sum  Inputs=|+++
  Terminator1 : Terminator
  u : Outport
  u1 : Outport  Port=2
  wires:
  errors/1 -> Demux/1
  Demux/1 -> Gain/1
  Demux/2 -> Gain1/1
  Demux/3 -> Gain2/1
  Demux/4 -> Gain3/1
  Sum/1 -> Gain5/1
  Gain3/1 -> Sum/4
  Gain2/1 -> Sum/3
  Gain1/1 -> Sum/2
  Gain/1 -> Sum/1
  errors1/1 -> Demux1/1
  PID Controller1/1 -> Gain4/1
  Demux1/4 -> Terminator1/1
  Gain4/1 -> u1/1, Scope2/1
  Gain5/1 -> u/1
  Demux1/2 -> Gain8/1
  Demux1/1 -> Saturation/1
  Demux1/3 -> Saturation1/1
  Sum1/1 -> PID Controller1/1
  Gain6/1 -> Sum1/2
  Gain7/1 -> Sum1/3
  Gain8/1 -> Sum1/1
  Saturation/1 -> Gain6/1
  Saturation1/1 -> Gain7/1

== system P1_Sim_2_1/another_try_with_control/not to escape watchdog ==
  In1 : Inport
  Sign : Signum
  l*cosx2 : Fcn  Expr=-u[1]
  Out1 : Outport
  wires:
  In1/1 -> l*cosx2/1
  l*cosx2/1 -> Sign/1
  Sign/1 -> Out1/1

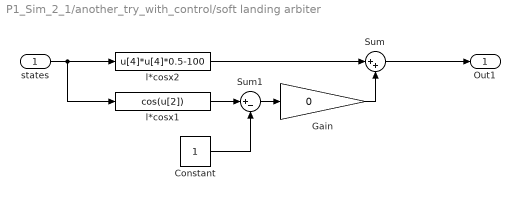
== system P1_Sim_2_1/another_try_with_control/soft landing arbiter ==
  states : Inport
  Constant : Constant
  Gain : Gain  Gain=0
  Sum : Sum  Inputs=|++
  Sum1 : Sum  Inputs=|+-
  l*cosx1 : Fcn  Expr=cos(u[2])
  l*cosx2 : Fcn  Expr=u[4]*u[4]*0.5-100
  Out1 : Outport
  wires:
  states/1 -> l*cosx1/1, l*cosx2/1
  l*cosx2/1 -> Sum/1
  Sum/1 -> Out1/1
  l*cosx1/1 -> Sum1/1
  Constant/1 -> Sum1/2
  Sum1/1 -> Gain/1
  Gain/1 -> Sum/2

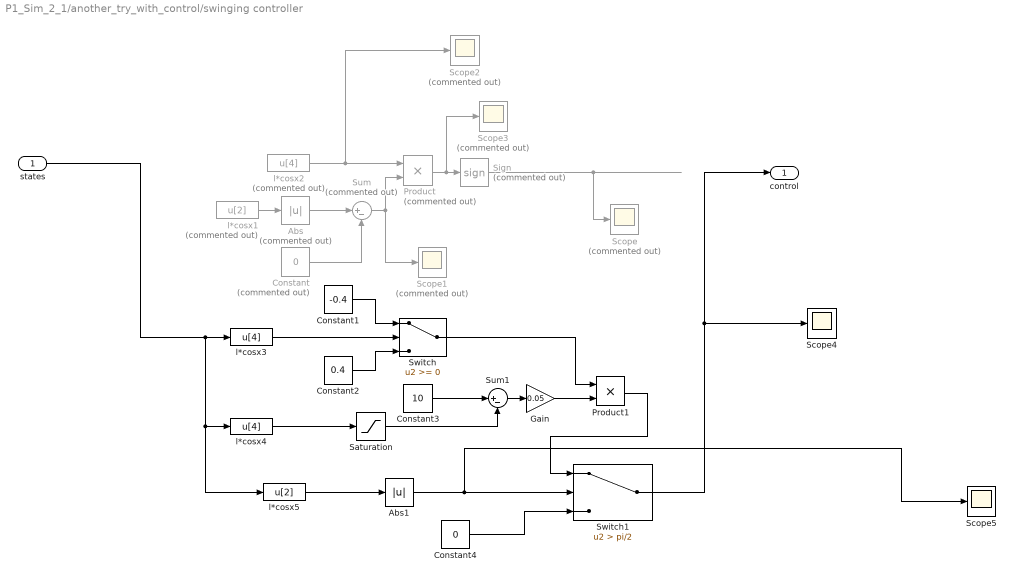
== system P1_Sim_2_1/another_try_with_control/swinging controller ==
  states : Inport
  Abs : Abs  Commented=on
  Abs1 : Abs
  Constant : Constant  Commented=on  Value=0
  Constant1 : Constant  Value=-0.4
  Constant2 : Constant  Value=0.4
  Constant3 : Constant  Value=10
  Constant4 : Constant  Value=0
  Gain : Gain  Gain=0.05
  Product : Product  Commented=on
  Product1 : Product
  Saturation : Saturate  UpperLimit=10  LowerLimit=-10
  Scope{,1..3} (4 alike) : Scope  Commented=on
  Scope4 : Scope
  Scope5 : Scope
  Sign : Signum  Commented=on
  Sum : Sum  Commented=on  Inputs=|+-
  Sum1 : Sum  Inputs=|+-
  Switch : Switch
  Switch1 : Switch  Criteria=u2 > Threshold  Threshold=pi/2
  l*cosx1 : Fcn  Commented=on  Expr=u[2]
  l*cosx2 : Fcn  Commented=on  Expr=u[4]
  l*cosx3 : Fcn  Expr=u[4]
  l*cosx4 : Fcn  Expr=u[4]
  l*cosx5 : Fcn  Expr=u[2]
  control : Outport
  wires:
  Product1/1 -> Switch1/1
  Abs1/1 -> Scope5/1, Switch1/2
  Switch/1 -> Product1/1
  Sum1/1 -> Gain/1
  Saturation/1 -> Sum1/2
  l*cosx4/1 -> Saturation/1
  Constant4/1 -> Switch1/3
  Constant3/1 -> Sum1/1
  Gain/1 -> Product1/2
  Switch1/1 -> control/1, Scope4/1
  l*cosx3/1 -> Switch/2
  Constant/1 -> Sum/2
  Sum/1 -> Scope1/1, Product/2
  l*cosx2/1 -> Scope2/1, Product/1
  Constant1/1 -> Switch/1
  l*cosx5/1 -> Abs1/1
  l*cosx1/1 -> Abs/1
  Product/1 -> Scope3/1, Sign/1
  states/1 -> l*cosx5/1, l*cosx4/1, l*cosx3/1
  Constant2/1 -> Switch/3
  Abs/1 -> Sum/1
  Sign/1 -> Scope/1

== system P1_Sim_2_1/another_try_with_control/upper zone arbiter ==
  In1 : Inport
  l*cosx2 : Fcn  Expr=abs(u[2])-pi/25
  Out1 : Outport
  wires:
  In1/1 -> l*cosx2/1
  l*cosx2/1 -> Out1/1

== matlab function P1_Sim_2_1/angle_convert ==
  data: angle_raw input; angle output
function angle = angle_convert(angle_raw)
    if angle_raw < 0
        is_negative = 1;
    else
        is_negative = 0;
    end
    if ~is_negative
        q = fix(angle_raw/2*pi);
        rem = mod(angle_raw,2*pi);
        if (rem >= pi && rem <= 2*pi)
            angle = -(2*pi - rem);
        else
            if q > 0
                angle = rem;
            else
                angle = angle_raw;
            end
        end
    else
        q = fix(-angle_raw/2*pi);
        rem = mod(-angle_raw,2*pi);
        if (rem >= pi && rem <= 2*pi)
            angle = (2*pi - rem);
        else
            if q > 0
                angle = -rem;
            else
                angle = angle_raw;
            end
        end
    end
end

== matlab function P1_Sim_2_1/angle_convert1 ==
  data: angle_raw input; angle output
function angle = angle_convert(angle_raw)
    if angle_raw < 0
        is_negative = 1;
    else
        is_negative = 0;
    end
    if ~is_negative
        q = fix(angle_raw/2*pi);
        rem = mod(angle_raw,2*pi);
        if (rem >= pi && rem <= 2*pi)
            angle = -(2*pi - rem);
        else
            if q > 0
                angle = rem;
            else
                angle = angle_raw;
            end
        end
    else
        q = fix(-angle_raw/2*pi);
        rem = mod(-angle_raw,2*pi);
        if (rem >= pi && rem <= 2*pi)
            angle = (2*pi - rem);
        else
            if q > 0
                angle = -rem;
            else
                angle = angle_raw;
            end
        end
    end
end
